simulink model "implementing_equations2"  (R2024a)
settings: Solver=VariableStepAuto  StartTime=0.0  StopTime=10.0  RelTol=1e-3
undefined symbols (not defined in the file or in its folder): ut
settings Model: Creator=robin  LastModifiedBy=robin

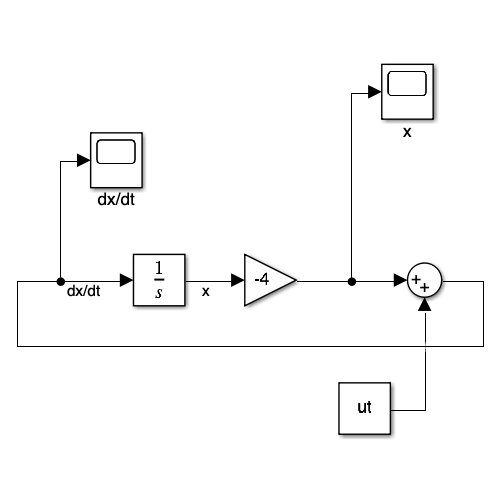
[thumbnail: Simulink's stored preview of the top-level diagram]
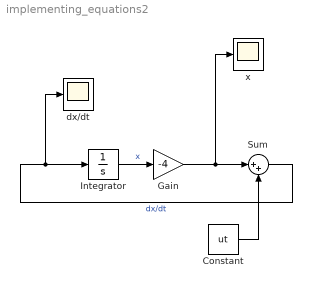
== system implementing_equations2 ==
  Constant : Constant  Value=ut
  Gain : Gain  Gain=-4
  Integrator : Integrator
  Sum : Sum  Inputs=|++
  dx/dt : Scope
  x : Scope
  wires:
  Sum/1 -> Integrator/1, dx/dt/1  "dx/dt"
  Integrator/1 -> Gain/1  "x"
  Constant/1 -> Sum/2
  Gain/1 -> x/1, Sum/1
